simulink model "ASD_current_source"  (R2021a)
settings: Solver=FixedStepAuto  StartTime=0.0  StopTime=0.5  FixedStep=1e-6  RelTol=1e-3
model workspace (MAT data in the model file):
  Sig = Simulink.Signal
  Sig.DataType = 'auto'
  Sig.Dimensions = -1
  Sig.DimensionsMode = 'auto'
  Sig.Complexity = 'auto'
  Sig.SampleTime = -1
  Sig.SamplingMode = 'auto'
  amplitue = 3
  freq = 400
libraries: spsIGBTDiodeLib x10, spsSeriesRLCBranchLib x4, spsCurrentMeasurementLib x2, spsThreePhaseSeriesRLCBranchLib x2, spsVoltageMeasurementLib x2, spsACVoltageSourceLib x1, spsAsynchronousMachineSIUnitsLib x1, autolibim x1, spsGroundLib x1, simulink x1, spsThreePhaseVIMeasurementLib x1, spspowerguiLib x1
settings Model: Creator=Mehra  LastModifiedBy=Mehra

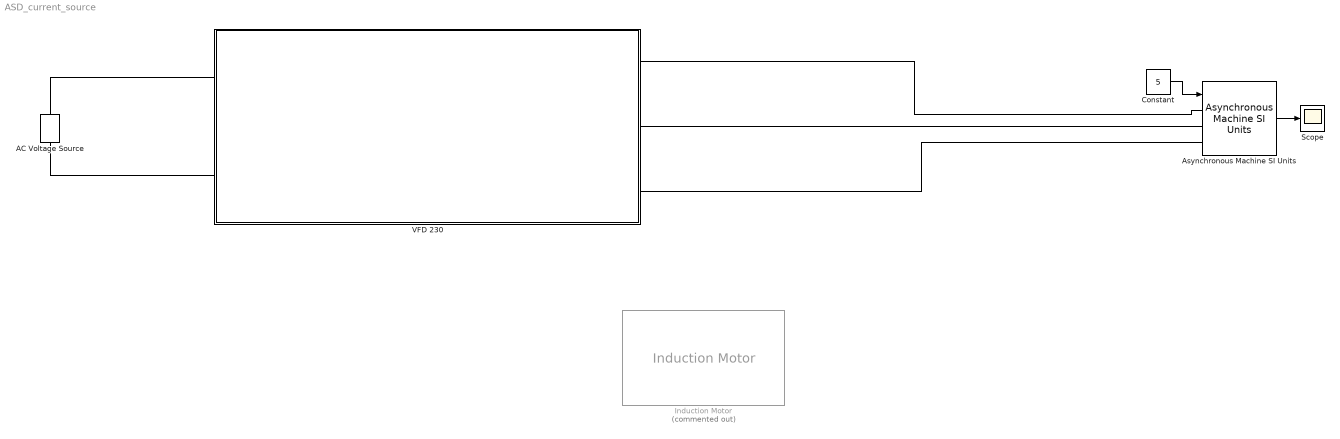
== system ASD_current_source ==
  AC Voltage Source : spsACVoltageSourceLib/AC Voltage Source  Amplitude=230  Phase=0  Frequency=60  SampleTime=0  Measurements=None  BusType=swing  Pref=10e3  Qref=0  Qmin=-inf  Qmax=+inf
  Asynchronous Machine SI Units : spsAsynchronousMachineSIUnitsLib/Asynchronous Machine SI Units  RotorType=Squirrel-cage  PresetModel=No  MechanicalLoad=Torque Tm  ShowDetailedParameters=on  ReferenceFrame=Rotor  Units=SI  MeasurementBus=off  NominalParameters=[1.845e+04 400 50]  VoltageRatio=1  Stator=[0.5968 0.0003495]  Rotor=[0.6258 0.005473]  Cage1=[0.4155 0.002066]  Cage2=[0.4168 0.0003495]  Lm=0.0354  Mechanical=[0.05 0.005879 2]  PolePairs=2  InitialConditions=[0 0 0 0 0 0 0 0]  SimulateSaturation=off  Saturation=[14.03593122, 27.81365428, 53.79336849, 72.68890987, 97.98006896, 148.6815601, 215.7428561, 302.9841135, 428.7778367 ; 230, 322, 414, 460, 506, 552, 598, 644, 690]  LoadFlowParameters=1492000  TsPowergui=0  TsBlock=-1  IterativeModel=Trapezoidal non iterative  IterativeDiscreteModel=Trapezoidal non iterative  Pmec=1.492e+006
  Constant : Constant  Value=5
  Induction Motor : autolibim/Induction Motor  Commented=on  sim_type=Continuous  Ts=0.001  port_config=Torque  P=2  Zs=[1.77 0.0139]  Zr="[1.34  0.0121]"  Lm=0.3687  mechanical=[0.001 0 0]  theta_init=0  omega_init=0  RefBlkName='autolibim/Induction Motor'  aMode=1
      settings: SourceProductBaseCode=PW,DR,MT,UV,VE
  Scope : Scope
  VFD 230 : Subsystem
  wires:
  Constant/1 -> Asynchronous Machine SI Units/1
  Asynchronous Machine SI Units/1 -> Scope/1
  connections:
  VFD 230/RConn1 -- Asynchronous Machine SI Units/LConn1
  Asynchronous Machine SI Units/LConn2 -- VFD 230/RConn2
  VFD 230/LConn1 -- AC Voltage Source/RConn1
  VFD 230/RConn3 -- Asynchronous Machine SI Units/LConn3
  VFD 230/LConn2 -- AC Voltage Source/LConn1

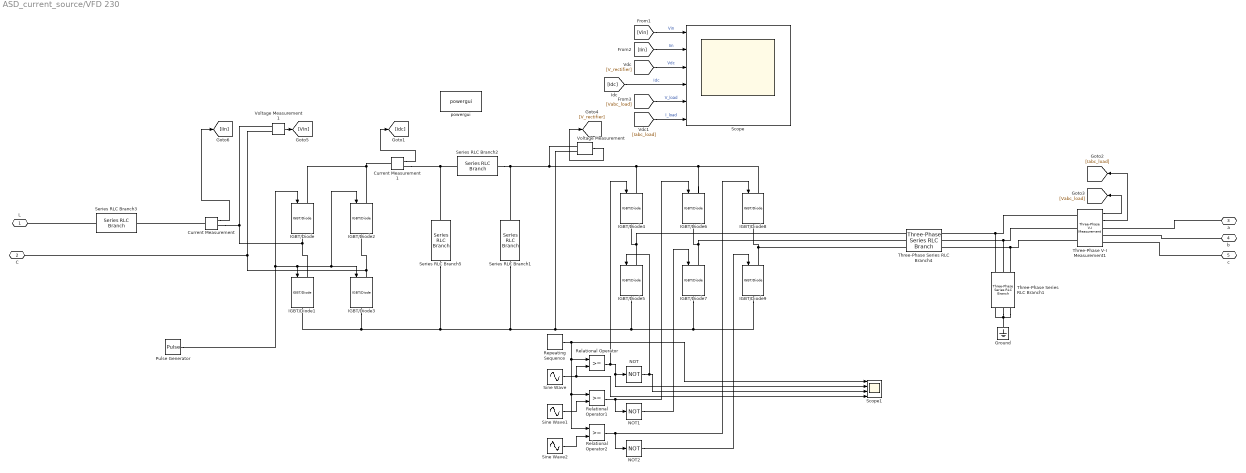
== system ASD_current_source/VFD 230 ==
  Current Measurement : spsCurrentMeasurementLib/Current Measurement  PhasorSimulation=off  OutputType=Complex  PSBequivalent=0
  Current Measurement1 : spsCurrentMeasurementLib/Current Measurement  PhasorSimulation=off  OutputType=Complex  PSBequivalent=0
  Ground : spsGroundLib/Ground  LConnTagsString=a
  IGBT/Diode{,1..9} (10 alike) : spsIGBTDiodeLib/IGBT//Diode  Ron=1e-3  Rs=1e5  Cs=inf  Measurements=off
  NOT : Logic  Operator=NOT  IconShape=distinctive  AllPortsSameDT=off  OutDataTypeStr=boolean
  NOT1 : Logic  Operator=NOT  IconShape=distinctive  AllPortsSameDT=off  OutDataTypeStr=boolean
  NOT2 : Logic  Operator=NOT  IconShape=distinctive  AllPortsSameDT=off  OutDataTypeStr=boolean
  Pulse Generator : DiscretePulseGenerator  PulseType=Time based  Period=0.0001  SampleTime=1e-5
  Relational Operator : RelationalOperator  OutDataTypeStr=boolean  RndMeth=Simplest
  Relational Operator1 : RelationalOperator  OutDataTypeStr=boolean  RndMeth=Simplest
  Relational Operator2 : RelationalOperator  OutDataTypeStr=boolean  RndMeth=Simplest
  Repeating Sequence : simulink/Sources/Repeating Sequence  rep_seq_t=[0 1/(freq*2000)]  rep_seq_y=[0 1]
  Scope : Scope  NumInputPorts=6
  Scope1 : Scope  NumInputPorts=4
  Series RLC Branch1 : spsSeriesRLCBranchLib/Series RLC Branch  LConnTagsString=__new0  RConnTagsString=__new0  BranchType=C  Resistance=10  Inductance=220e-6  SetiL0=off  InitialCurrent=0  Capacitance=240e-6  Setx0=off  InitialVoltage=0  Measurements=Branch current
  Series RLC Branch2 : spsSeriesRLCBranchLib/Series RLC Branch  LConnTagsString=__new0  RConnTagsString=__new0  BranchType=L  Resistance=10  Inductance=470e-6  SetiL0=off  InitialCurrent=0  Capacitance=47e-6  Setx0=off  InitialVoltage=0  Measurements=Branch current
  Series RLC Branch3 : spsSeriesRLCBranchLib/Series RLC Branch  LConnTagsString=__new0  RConnTagsString=__new0  BranchType=L  Resistance=10  Inductance=470e-6  SetiL0=off  InitialCurrent=0  Capacitance=47e-6  Setx0=off  InitialVoltage=0  Measurements=Branch current
  Series RLC Branch5 : spsSeriesRLCBranchLib/Series RLC Branch  LConnTagsString=__new0  RConnTagsString=__new0  BranchType=C  Resistance=10  Inductance=220e-6  SetiL0=off  InitialCurrent=0  Capacitance=240e-6  Setx0=off  InitialVoltage=0  Measurements=Branch current
  Sine Wave : Sin  Amplitude=amplitue  Frequency=2*pi*freq  SampleTime=1e-5
  Sine Wave1 : Sin  Amplitude=amplitue  Frequency=2*pi*freq  Phase=2*pi/3  SampleTime=1e-5
  Sine Wave2 : Sin  Amplitude=amplitue  Frequency=2*pi*freq  Phase=4*pi/3  SampleTime=1e-5
  Three-Phase Series RLC Branch1 : spsThreePhaseSeriesRLCBranchLib/Three-Phase Series RLC Branch  LConnTagsString=A|B|C  RConnTagsString=A|B|C  BranchType=C  Resistance=1  Inductance=470e-6  Capacitance=200e-6  Measurements=None
  Three-Phase Series RLC Branch4 : spsThreePhaseSeriesRLCBranchLib/Three-Phase Series RLC Branch  LConnTagsString=A|B|C  RConnTagsString=A|B|C  BranchType=L  Resistance=1  Inductance=470e-6  Capacitance=470e-6  Measurements=None
  Three-Phase V-I Measurement1 : spsThreePhaseVIMeasurementLib/Three-Phase V-I Measurement  VoltageMeasurement=phase-to-ground  SetLabelV=off  LabelV=Vabc  Vpu=off  VpuLL=off  CurrentMeasurement=yes  SetLabelI=off  LabelI=Iabc  Ipu=off  Pbase=100e6  Vbase=500e3  OutputType=Complex  PhasorSimulation=off  PSBequivalent=0
  Voltage Measurement : spsVoltageMeasurementLib/Voltage Measurement  PhasorSimulation=off  OutputType=Complex  PSBequivalent=0
  Voltage Measurement1 : spsVoltageMeasurementLib/Voltage Measurement  PhasorSimulation=off  OutputType=Complex  PSBequivalent=0
  powergui : spspowerguiLib/powergui  Priority=1  SimulationMode=Discrete  SampleTime=1e-6  frequency=60  Iterations=50  frequencyindice=0  Pbase=100e6  ErrMax=1e-4  UnitsV=kV  UnitsW=MW  buscounter=0  FunctionMessages=off  echomessages=off  EnableUseOfTLC=off  CurrentSourceSwitches=off  DisableSnubberDevices=off  DisableRonSwitches=off  DisableVfSwitches=off  DisplayEquations=off  AutomaticDiscreteSolvers=off  SolverType=Tustin/Backward Euler (TBE)  Interpol=off  ExternalGateDelay=off  methode=off  Ts=100  x0status=blocks  SPID=on  SwTol=0  HookPort=off  NonlinearTolerance=1e-4  nMaxIteration=100  ContinueOnMaxIteration=off  RestoreLinks=warning  ResistiveCurrentMeasurement=off  Frange=[0:2:500]  Ylog=off  Xlog=on  ShowGrid=off  save=off  variable=ZData  structure=0  ZoomFFT=off  StartTime=0.0  cycles=1  DisplayStyle=1  fundamental=60  FreqAxis=off  MaxFrequency=1000  frequencyindicesteady=1  RmsSteady=1  display=off
  L : PMIOPort  Side=Left
  C : PMIOPort  Port=2  Side=Left
  a : PMIOPort  Port=3  Side=Right
  b : PMIOPort  Port=4  Side=Right
  c : PMIOPort  Port=5  Side=Right
  wires:
  Voltage Measurement1/1 -> [Vin]
  Relational Operator1/1 -> IGBT/Diode6/1, NOT1/1
  [Iin] -> Scope/2  "Iin"
  Relational Operator/1 -> Scope1/2, NOT/1, IGBT/Diode4/1
  Sine Wave/1 -> Scope1/4, Relational Operator/2
  Current Measurement1/1 -> [Idc]
  Three-Phase V-I Measurement1/2 -> [Iabc_load]
  Repeating Sequence/1 -> Relational Operator2/1, Relational Operator1/1, Relational Operator/1, Scope1/1
  NOT2/1 -> IGBT/Diode9/1
  [Vabc_load] -> Scope/5  "V_load"
  Sine Wave1/1 -> Relational Operator1/2
  Three-Phase V-I Measurement1/1 -> [Vabc_load]
  NOT/1 -> Scope1/3, IGBT/Diode5/1
  NOT1/1 -> IGBT/Diode7/1
  [Iabc_load] -> Scope/6  "I_load"
  [V_rectifier] -> Scope/3  "Vdc"
  Voltage Measurement/1 -> [V_rectifier]
  [Vin] -> Scope/1  "Vin"
  [Idc] -> Scope/4  "Idc"
  Relational Operator2/1 -> IGBT/Diode8/1, NOT2/1
  Pulse Generator/1 -> IGBT/Diode/1, IGBT/Diode2/1, IGBT/Diode3/1, IGBT/Diode1/1
  Current Measurement/1 -> [Iin]
  Sine Wave2/1 -> Relational Operator2/2
  connections:
  IGBT/Diode9/LConn1 -- IGBT/Diode8/RConn1 -- Three-Phase Series RLC Branch4/LConn3
  Voltage Measurement/LConn2 -- IGBT/Diode9/RConn1 -- IGBT/Diode7/RConn1 -- IGBT/Diode5/RConn1 -- Series RLC Branch1/RConn1 -- Series RLC Branch5/RConn1 -- IGBT/Diode3/RConn1 -- IGBT/Diode1/RConn1
  Series RLC Branch5/LConn1 -- Series RLC Branch2/RConn1 -- Current Measurement1/RConn1
  Three-Phase V-I Measurement1/LConn2 -- Three-Phase Series RLC Branch1/LConn2 -- Three-Phase Series RLC Branch4/RConn2
  Series RLC Branch2/LConn1 -- Series RLC Branch1/LConn1 -- Voltage Measurement/LConn1 -- IGBT/Diode8/LConn1 -- IGBT/Diode6/LConn1 -- IGBT/Diode4/LConn1
  IGBT/Diode7/LConn1 -- Three-Phase Series RLC Branch4/LConn2 -- IGBT/Diode6/RConn1
  IGBT/Diode/LConn1 -- IGBT/Diode2/LConn1 -- Current Measurement1/LConn1
  Ground/LConn1 -- Three-Phase Series RLC Branch1/RConn1 -- Three-Phase Series RLC Branch1/RConn3 -- Three-Phase Series RLC Branch1/RConn2
  Three-Phase V-I Measurement1/LConn1 -- Three-Phase Series RLC Branch4/RConn1 -- Three-Phase Series RLC Branch1/LConn1
  IGBT/Diode5/LConn1 -- Three-Phase Series RLC Branch4/LConn1 -- IGBT/Diode4/RConn1
  Current Measurement/LConn1 -- Series RLC Branch3/LConn1
  IGBT/Diode/RConn1 -- Voltage Measurement1/LConn1 -- Current Measurement/RConn1 -- IGBT/Diode1/LConn1
  b/RConn1 -- Three-Phase V-I Measurement1/RConn2
  Three-Phase V-I Measurement1/LConn3 -- Three-Phase Series RLC Branch1/LConn3 -- Three-Phase Series RLC Branch4/RConn3
  IGBT/Diode2/RConn1 -- Voltage Measurement1/LConn2 -- C/RConn1 -- IGBT/Diode3/LConn1
  a/RConn1 -- Three-Phase V-I Measurement1/RConn1
  c/RConn1 -- Three-Phase V-I Measurement1/RConn3
  Series RLC Branch3/RConn1 -- L/RConn1
